simulink model "main_sim5"  (R2023a)
settings: Solver=FixedStepAuto  StartTime=0.0  StopTime=T  FixedStep=dt  RelTol=1e-3
values from neighbouring files (symbols this model uses):
  A = -a * eye(4)    [main_real4_slx.m]    (also in main_sim5_slx.m)
  ctrl_dt = 2e-3    (= 0.002)    [main_real4_slx.m]    (also in main_sim5_slx.m = 0.001)
  dt = time(2) - time(1)    [check_PE_from_logsout.m]    (also in main_real4_slx.m = 0.002; main_sim5_slx.m = 0.001)
  eta1 = 1e3    (= 1000)    [main_real4_slx.m]    (also in main_sim5_slx.m = 0.1)
  eta2 = 1e2    (= 100)    [main_real4_slx.m]    (also in main_sim5_slx.m)
  Kd = [20 0 ... (first row only)    [main_real4_slx.m]    (also in main_sim5_slx.m)
  Kp = [100 0 ... (first row only)    [main_real4_slx.m]    (also in main_sim5_slx.m)
  N = length(time)    [check_PE_from_logsout.m]    (also in main_plotter5_1.m = length(X3); main_plotter5_2.m = length(X3))
  n_h = 100    [main_real4_slx.m]    (also in main_sim5_slx.m = 20)
  n_i = 6    [main_real4_slx.m]    (also in main_sim5_slx.m)
  n_o = 4    [main_real4_slx.m]    (also in main_sim5_slx.m)
  params = struct(     'm1', 2.465,     'm2', 2.465,     'l1', 0.2,     'l2', 0.2,     'lc1', 0.13888,     'lc2', 0.13888,     'I1', 0.06911,     'I2', 0.06911,     'I1m', 9*9*1002e-7,     'I2m', 9*9*1002e-7,     'b1', 0.5,     'b2', 0.7,     'fc1', 0.1,     'fc2', 0.1,     'k1', 1500,     'k2', 1500)    [main_real4_slx.m]    (also in main_sim5_slx.m = struct(     'm1', 2.465,     'm2', 2.465,     'l1', 0.2,    )
  rho1 = 0.0    (= 0)    [main_real4_slx.m]    (also in main_sim5_slx.m)
  rho2 = 0.0    (= 0)    [main_real4_slx.m]    (also in main_sim5_slx.m)
  V0 = 1e-2 * randn(n_h,n_i) + 0    [main_real4_slx.m]    (also in main_sim5_slx.m = 1e-1 * randn(n_h,n_i))
  W0 = 1e-2 * randn(n_o,n_h) + 0    [main_real4_slx.m]    (also in main_sim5_slx.m = 1e-1 * randn(n_o,n_h))
  X0 = [data_2901(1,1);data_2902(1,1);data_2901(2,1);data_2902(2,1)]    [main_real4_slx.m]    (also in main_sim5_slx.m = [-pi/2; 0; 0; 0])
  X_hat_0 = X0    [main_real4_slx.m]    (also in main_sim5_slx.m)
undefined symbols (not defined in the file or in its folder): I1, I1m, I2, I2m, J_V_t_buffer, J_W_t_buffer, l1, l2, lc1, lc2, m1, m2
settings Model: Creator=dding  LastModifiedBy=fairytale

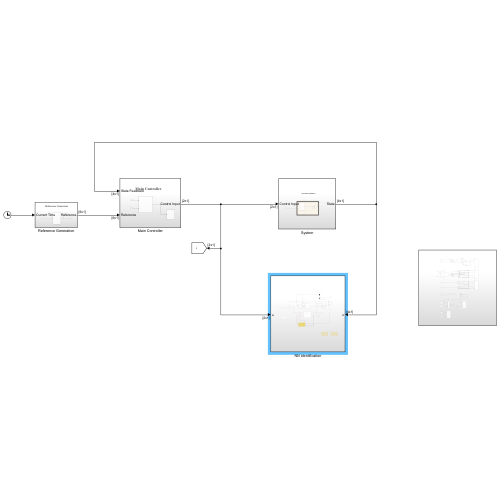
[thumbnail: Simulink's stored preview of the top-level diagram]
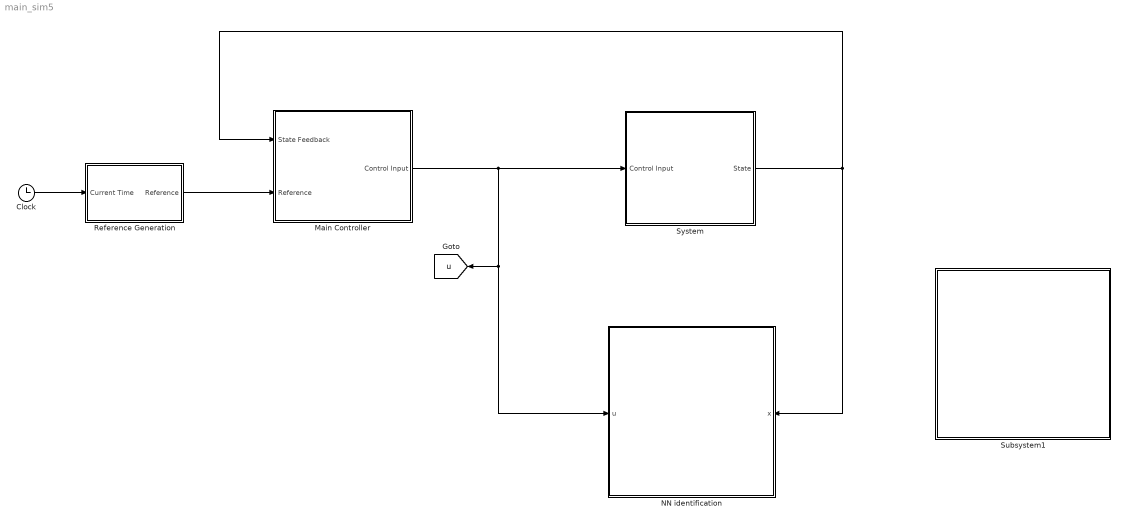
== system main_sim5 ==
  Clock : Clock
  Main Controller : Subsystem
  NN identification : Subsystem
      settings: PortSchema="{\"entries\":[{\"content\":{\"sides\":[{\"content\":{},\"type\":\"ConnectorPlacement.EquallySpacedRectSide\",\"uuid\":\"b5e68509-af14-483e-9022-a238da7f8976\"},{\"content\":{\"side\":\"RIGHT\"},\"type\":\"ConnectorPlacement.EquallySpacedRectSide\",\"uuid\":\"227b12d5-85c0-4871-b1f3-ce700a25cbd8\"},{\"content\":{\"connectorIds\":[\"In1\"],\"side\":\"TOP\"},\"type\":\"ConnectorPlacement.EquallySpacedRectSide\",\"uuid\":\"04532d91-bd13-4081-a0a6-2e9b5f5bbbc1\"},{\"content\":{\"connectorIds\":[\"In2\"],\"side\":\"BOTTOM\"},\"type\":\"ConnectorPlacement.EquallySpacedRectSide\",\"uuid\":\"58e23698-c698-43c7-afbb-9eb032c0630e\"}]},\"type\":\"ConnectorPlacement.EquallySpacedConnector\",\"uuid\":\"69e78e49-5ac8-44ff-82c8-e58de664d9c5\"}],\"packageUris\":[\"http://schema.mathworks.com/mf0/Connector/R2020b\"],\"version\":\"1.0\"}"
  Reference Generation : Subsystem
  Subsystem1 : Subsystem
  System : Subsystem
  tag scope: u=global
  wires:
  Reference Generation/1(Reference) -> Main Controller/2(Reference)
  Clock/1 -> Reference Generation/1(Current Time)
  Main Controller/1(Control Input) -> System/1(Control Input), NN identification/1(u), [u]
  System/1(State) -> NN identification/2(x), Main Controller/1(State Feedback)

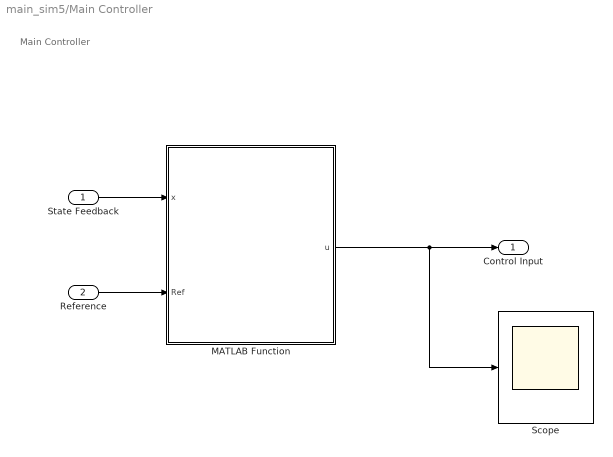
== system main_sim5/Main Controller ==
  note: Main Controller
  State Feedback : Inport
  Reference : Inport  Port=2
  MATLAB Function : MATLAB Function  TreatAsAtomicUnit=on  SystemSampleTime=ctrl_dt
  Scope : Scope
  Control Input : Outport
  wires:
  Reference/1 -> MATLAB Function/2(Ref)
  State Feedback/1 -> MATLAB Function/1(x)
  MATLAB Function/1(u) -> Scope/1, Control Input/1

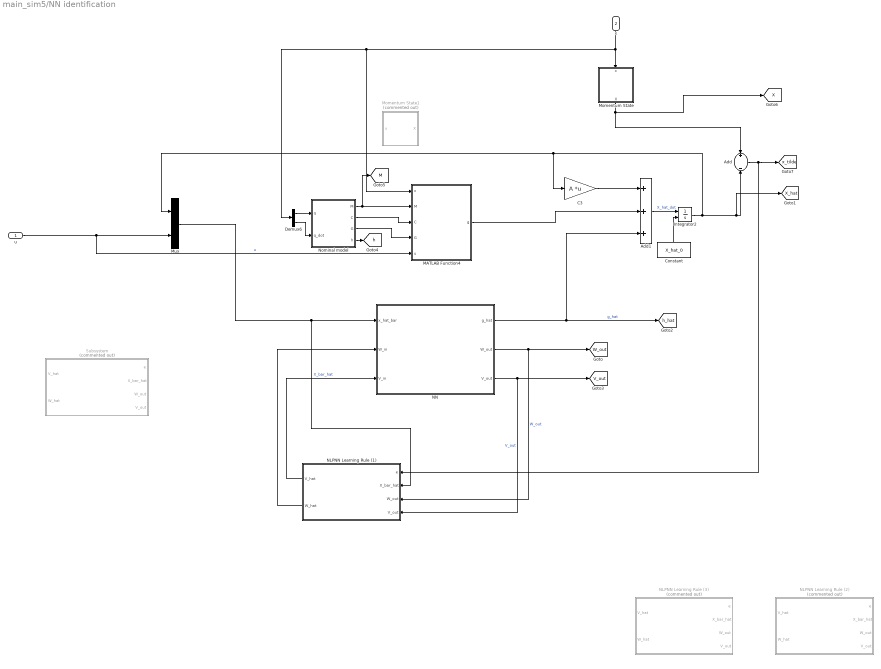
== system main_sim5/NN identification ==
  u : Inport
  x : Inport  Port=2
  Add : Sum  Inputs=+-
  Add1 : Sum  Inputs=+++
  C3 : Gain  Gain=A  Multiplication=Matrix(K*u)
  Constant : Constant  Value=X_hat_0  VectorParams1D=off
  Demux6 : Demux  Outputs=2
  Integrator2 : Integrator  InitialConditionSource=external  InitialCondition=X_hat_0
  MATLAB Function4 : MATLAB Function  TreatAsAtomicUnit=on
  Momentum State : MATLAB Function  TreatAsAtomicUnit=on
  Momentum State1 : MATLAB Function  Commented=on  TreatAsAtomicUnit=on
  Mux : Mux  Inputs=2
  NLPNN Learning Rule (1) : Subsystem
  NLPNN Learning Rule (2) : Subsystem  Commented=on
  NLPNN Learning Rule (3) : Subsystem  Commented=on
  NN : MATLAB Function  TreatAsAtomicUnit=on
  Nominal model : MATLAB Function  TreatAsAtomicUnit=on
  Subsystem : Subsystem  Commented=on
  tag scope: M=global, V_out=global, W_out=global, X=global, X_hat=global, h=global, h_hat=global, x_tilde=global
  wires:
  x/1 -> Demux6/1, MATLAB Function4/1(x), Momentum State/1(x)
  NN/2(W_out) -> NLPNN Learning Rule (1)/3(W_out), [W_out]  "W_out"
  Integrator2/1 -> Add/2, [X_hat], C3/1, Mux/1
  Add1/1 -> Integrator2/1  "X_hat_dot"
  NN/3(V_out) -> NLPNN Learning Rule (1)/4(V_out), [V_out]  "V_out"
  u/1 -> MATLAB Function4/5(u), Mux/2  "u"
  C3/1 -> Add1/1
  NN/1(g_hat) -> [h_hat], Add1/3  "g_hat"
  Constant/1 -> Integrator2/2
  Mux/1 -> NLPNN Learning Rule (1)/2(X_bar_hat), NN/1(x_hat_bar)  "X_bar_hat"
  Demux6/1 -> Nominal model/1(q)
  Nominal model/1(M) -> MATLAB Function4/2(M), [M]
  Nominal model/3(G) -> MATLAB Function4/4(G)
  Nominal model/2(C) -> MATLAB Function4/3(C)
  Demux6/2 -> Nominal model/2(q_dot)
  Momentum State/1(X) -> [X], Add/1
  Nominal model/4(h) -> [h]
  Add/1 -> NLPNN Learning Rule (1)/1(e), [x_tilde]
  NLPNN Learning Rule (1)/1(V_hat) -> NN/3(V_in)
  NLPNN Learning Rule (1)/2(W_hat) -> NN/2(W_in)
  MATLAB Function4/1(g) -> Add1/2

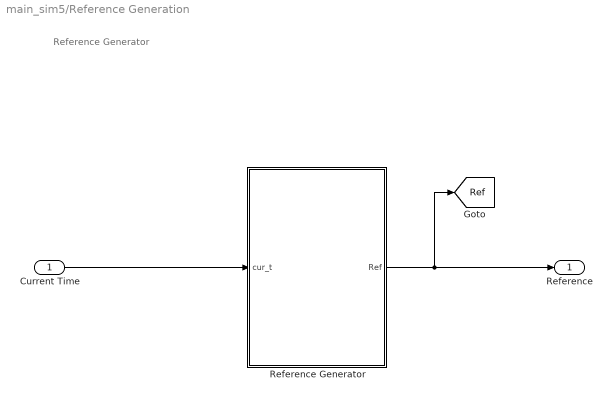
== system main_sim5/Reference Generation ==
  note: Reference Generator
  Current Time : Inport
  Reference Generator : MATLAB Function  TreatAsAtomicUnit=on
  Reference : Outport
  tag scope: Ref=global
  wires:
  Current Time/1 -> Reference Generator/1(cur_t)
  Reference Generator/1(Ref) -> [Ref], Reference/1

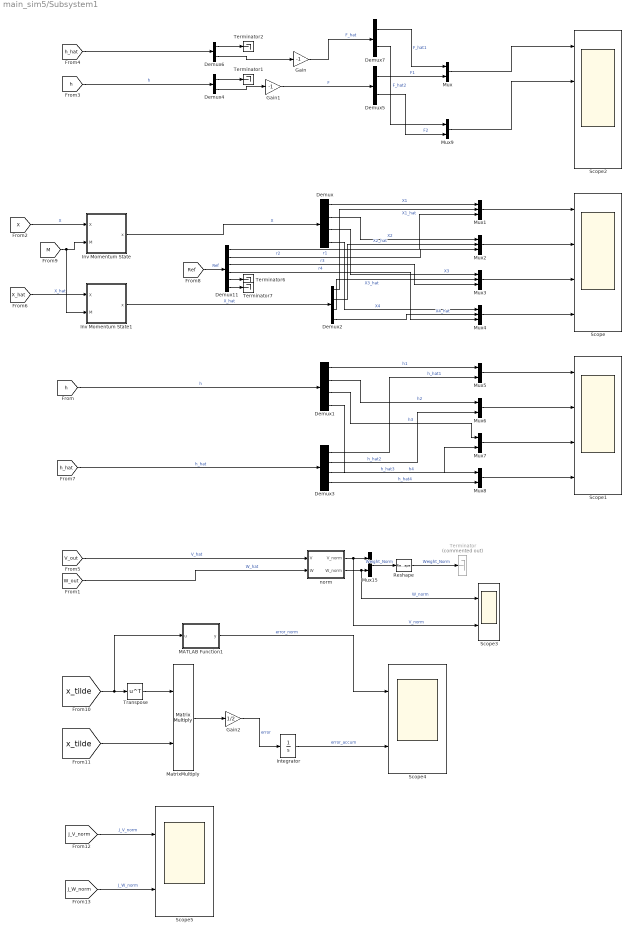
== system main_sim5/Subsystem1 ==
  Demux{,1..3} (4 alike) : Demux
  Demux11 : Demux  Outputs=6
  Demux{4..7} (4 alike) : Demux  Outputs=2
  Gain : Gain  Gain=-1
  Gain1 : Gain  Gain=-1
  Gain2 : Gain  Gain=1/2
  Integrator : Integrator
  Inv Momentum State : MATLAB Function  TreatAsAtomicUnit=on
  Inv Momentum State1 : MATLAB Function  TreatAsAtomicUnit=on
  MATLAB Function1 : MATLAB Function  TreatAsAtomicUnit=on
  MatrixMultiply : Product  Multiplication=Matrix(*)
  Mux{,5..9,15} (7 alike) : Mux  Inputs=2
  Mux{1..4} (4 alike) : Mux  Inputs=3
  Reshape : Reshape  OutputDimensionality=Column vector (2-D)
  Scope : Scope  NumInputPorts=4
  Scope1 : Scope  NumInputPorts=4
  Scope2 : Scope  NumInputPorts=4
  Scope3 : Scope  NumInputPorts=2
  Scope4 : Scope  NumInputPorts=2
  Scope5 : Scope  NumInputPorts=2
  Terminator : Terminator  Commented=on
  Terminator{1..2,6..7} (4 alike) : Terminator
  Transpose : Math  Operator=transpose
  norm : MATLAB Function  TreatAsAtomicUnit=on
  wires:
  Demux2/2 -> Mux2/2  "X2_hat"
  Mux4/1 -> Scope/4
  Demux1/4 -> Mux8/1  "h4"
  Mux3/1 -> Scope/3
  [h_hat] -> Demux3/1  "h_hat"
  Demux3/1 -> Mux5/2  "h_hat1"
  Demux3/2 -> Mux6/2  "h_hat2"
  Demux/1 -> Mux1/1  "X1"
  [Ref] -> Demux11/1  "Ref"
  Mux5/1 -> Scope1/1
  Demux1/1 -> Mux5/1  "h1"
  Mux2/1 -> Scope/2
  Demux2/4 -> Mux4/2  "X4_hat"
  Demux/3 -> Mux3/1  "X3"
  Demux11/1 -> Mux1/3  "r1"
  Mux6/1 -> Scope1/2
  Demux11/3 -> Mux3/3  "r3"
  Demux11/2 -> Mux2/3  "r2"
  Mux7/1 -> Scope1/3
  Demux2/1 -> Mux1/2  "X1_hat"
  Mux8/1 -> Scope1/4
  Demux2/3 -> Mux3/2  "X3_hat"
  Demux/4 -> Mux4/1  "X4"
  Demux11/6 -> Terminator7/1
  Demux/2 -> Mux2/1  "X2"
  Mux1/1 -> Scope/1
  Demux3/4 -> Mux8/2  "h_hat4"
  Demux11/5 -> Terminator6/1
  [h_hat] -> Demux6/1
  Demux1/2 -> Mux6/1  "h2"
  Demux3/3 -> Mux7/2  "h_hat3"
  Demux1/3 -> Mux7/1  "h3"
  [h] -> Demux1/1  "h"
  Demux11/4 -> Mux4/3  "r4"
  Demux5/1 -> Mux/2  "F1"
  Demux5/2 -> Mux9/2  "F2"
  norm/1(V_norm) -> Scope3/2, Mux15/1  "V_norm"
  Reshape/1 -> Terminator/1  "Weight_Norm"
  norm/2(W_norm) -> Scope3/1, Mux15/2  "W_norm"
  Mux15/1 -> Reshape/1  "Weight_Norm"
  [W_out] -> norm/2(W)  "W_hat"
  [V_out] -> norm/1(V)  "V_hat"
  [h] -> Demux4/1  "h"
  Demux4/1 -> Terminator1/1
  Demux6/1 -> Terminator2/1
  Demux6/2 -> Gain/1
  Demux4/2 -> Gain1/1
  Gain1/1 -> Demux5/1  "F"
  Gain/1 -> Demux7/1  "F_hat"
  Demux7/1 -> Mux/1  "F_hat1"
  Demux7/2 -> Mux9/1  "F_hat2"
  Mux/1 -> Scope2/1
  Mux9/1 -> Scope2/2
  [X] -> Inv Momentum State/1(X)  "X"
  [X_hat] -> Inv Momentum State1/1(X)  "X_hat"
  Inv Momentum State/1(x) -> Demux/1  "X"
  Inv Momentum State1/1(x) -> Demux2/1  "X_hat"
  [M] -> Inv Momentum State1/2(M), Inv Momentum State/2(M)
  [x_tilde] -> MATLAB Function1/1(u), Transpose/1
  Transpose/1 -> MatrixMultiply/1
  [x_tilde] -> MatrixMultiply/2
  MatrixMultiply/1 -> Gain2/1
  Gain2/1 -> Integrator/1  "error"
  Integrator/1 -> Scope4/2  "error_accum"
  [J_V_norm] -> Scope5/1  "J_V_norm"
  [J_W_norm] -> Scope5/2  "J_W_norm"
  MATLAB Function1/1(y) -> Scope4/1  "error_norm"

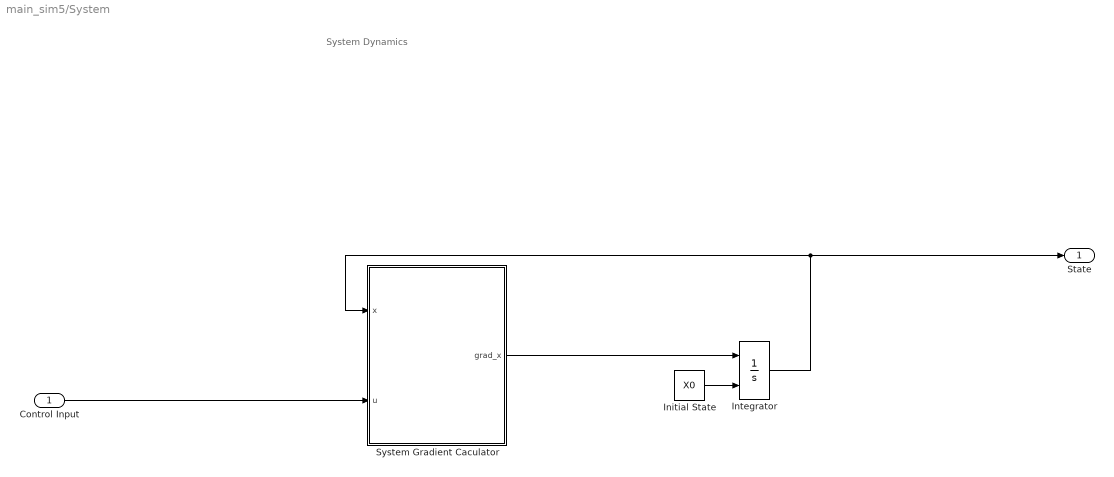
== system main_sim5/System ==
  note: System Dynamics
  Control Input : Inport
  Initial State : Constant  Value=X0  VectorParams1D=off
  Integrator : Integrator  InitialConditionSource=external
  System Gradient Caculator : MATLAB Function  TreatAsAtomicUnit=on
  State : Outport
  wires:
  Initial State/1 -> Integrator/2
  Control Input/1 -> System Gradient Caculator/2(u)
  Integrator/1 -> System Gradient Caculator/1(x), State/1
  System Gradient Caculator/1(grad_x) -> Integrator/1

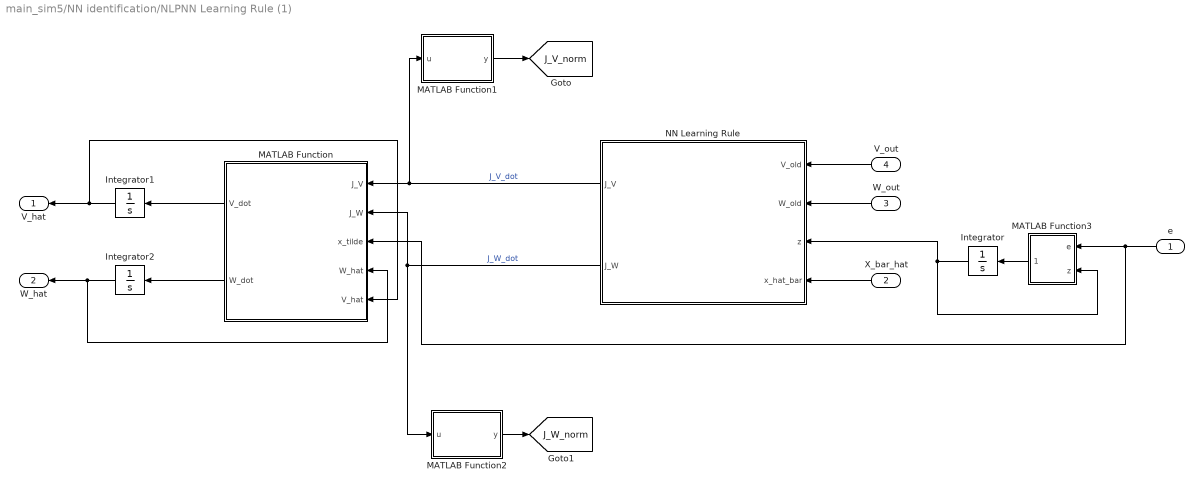
== system main_sim5/NN identification/NLPNN Learning Rule (1) ==
  e : Inport
  X_bar_hat : Inport  Port=2
  W_out : Inport  Port=3
  V_out : Inport  Port=4
  Integrator : Integrator  InitialCondition=[0,0,0,0]'
  Integrator1 : Integrator  InitialCondition=V0
  Integrator2 : Integrator  InitialCondition=W0
  MATLAB Function : MATLAB Function  TreatAsAtomicUnit=on
  MATLAB Function1 : MATLAB Function  TreatAsAtomicUnit=on
  MATLAB Function2 : MATLAB Function  TreatAsAtomicUnit=on
  MATLAB Function3 : MATLAB Function  TreatAsAtomicUnit=on
  NN Learning Rule : MATLAB Function  TreatAsAtomicUnit=on
  V_hat : Outport
  W_hat : Outport  Port=2
  tag scope: J_V_norm=global, J_W_norm=global
  wires:
  e/1 -> MATLAB Function/3(x_tilde), MATLAB Function3/1(e)
  X_bar_hat/1 -> NN Learning Rule/4(x_hat_bar)
  W_out/1 -> NN Learning Rule/2(W_old)
  V_out/1 -> NN Learning Rule/1(V_old)
  MATLAB Function/1(V_dot) -> Integrator1/1
  Integrator1/1 -> MATLAB Function/5(V_hat), V_hat/1
  Integrator2/1 -> MATLAB Function/4(W_hat), W_hat/1
  MATLAB Function/2(W_dot) -> Integrator2/1
  MATLAB Function1/1(y) -> [J_V_norm]
  MATLAB Function2/1(y) -> [J_W_norm]
  MATLAB Function3/1(z_dot) -> Integrator/1
  NN Learning Rule/2(J_W) -> MATLAB Function2/1(u), MATLAB Function/2(J_W)  "J_W_dot"
  NN Learning Rule/1(J_V) -> MATLAB Function1/1(u), MATLAB Function/1(J_V)  "J_V_dot"
  Integrator/1 -> MATLAB Function3/2(z), NN Learning Rule/3(z)

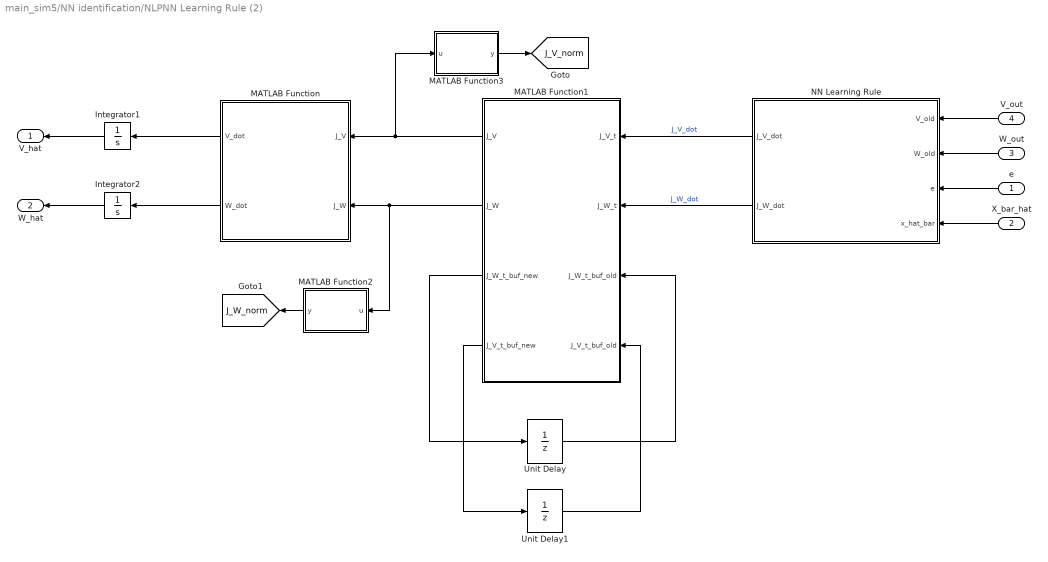
== system main_sim5/NN identification/NLPNN Learning Rule (2) ==
  e : Inport
  X_bar_hat : Inport  Port=2
  W_out : Inport  Port=3
  V_out : Inport  Port=4
  Integrator1 : Integrator  InitialCondition=V0
  Integrator2 : Integrator  InitialCondition=W0
  MATLAB Function : MATLAB Function  TreatAsAtomicUnit=on
  MATLAB Function1 : MATLAB Function  TreatAsAtomicUnit=on
  MATLAB Function2 : MATLAB Function  TreatAsAtomicUnit=on
  MATLAB Function3 : MATLAB Function  TreatAsAtomicUnit=on
  NN Learning Rule : MATLAB Function  TreatAsAtomicUnit=on
  Unit Delay : UnitDelay  InitialCondition=J_W_t_buffer  SampleTime=-1  HasFrameUpgradeWarning=on
  Unit Delay1 : UnitDelay  InitialCondition=J_V_t_buffer  SampleTime=-1  HasFrameUpgradeWarning=on
  V_hat : Outport
  W_hat : Outport  Port=2
  tag scope: J_V_norm=global, J_W_norm=global
  wires:
  e/1 -> NN Learning Rule/3(e)
  X_bar_hat/1 -> NN Learning Rule/4(x_hat_bar)
  W_out/1 -> NN Learning Rule/2(W_old)
  V_out/1 -> NN Learning Rule/1(V_old)
  NN Learning Rule/1(J_V_dot) -> MATLAB Function1/1(J_V_t)  "J_V_dot"
  NN Learning Rule/2(J_W_dot) -> MATLAB Function1/2(J_W_t)  "J_W_dot"
  MATLAB Function/1(V_dot) -> Integrator1/1
  Integrator1/1 -> V_hat/1
  Integrator2/1 -> W_hat/1
  MATLAB Function/2(W_dot) -> Integrator2/1
  MATLAB Function1/1(J_V) -> MATLAB Function3/1(u), MATLAB Function/1(J_V)
  MATLAB Function1/2(J_W) -> MATLAB Function2/1(u), MATLAB Function/2(J_W)
  Unit Delay/1 -> MATLAB Function1/3(J_W_t_buf_old)
  MATLAB Function1/3(J_W_t_buf_new) -> Unit Delay/1
  MATLAB Function1/4(J_V_t_buf_new) -> Unit Delay1/1
  Unit Delay1/1 -> MATLAB Function1/4(J_V_t_buf_old)
  MATLAB Function2/1(y) -> [J_W_norm]
  MATLAB Function3/1(y) -> [J_V_norm]

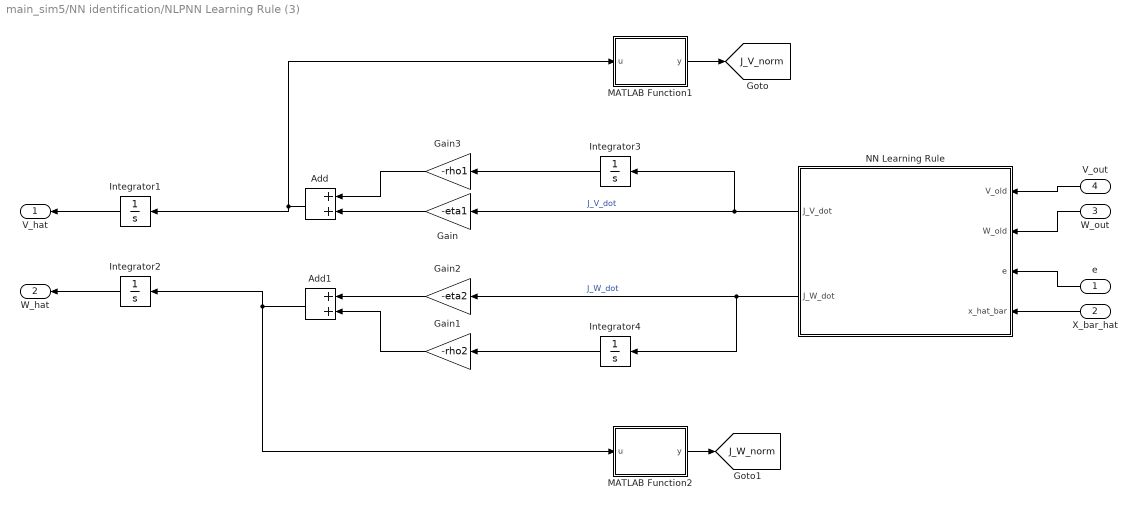
== system main_sim5/NN identification/NLPNN Learning Rule (3) ==
  e : Inport
  X_bar_hat : Inport  Port=2
  W_out : Inport  Port=3
  V_out : Inport  Port=4
  Add : Sum
  Add1 : Sum
  Gain : Gain  Gain=-eta1
  Gain1 : Gain  Gain=-rho2
  Gain2 : Gain  Gain=-eta2
  Gain3 : Gain  Gain=-rho1
  Integrator1 : Integrator  InitialCondition=V0
  Integrator2 : Integrator  InitialCondition=W0
  Integrator3 : Integrator  InitialCondition=zeros(n_h,n_i)
  Integrator4 : Integrator  InitialCondition=zeros(n_o,n_h)
  MATLAB Function1 : MATLAB Function  TreatAsAtomicUnit=on
  MATLAB Function2 : MATLAB Function  TreatAsAtomicUnit=on
  NN Learning Rule : MATLAB Function  TreatAsAtomicUnit=on
  V_hat : Outport
  W_hat : Outport  Port=2
  tag scope: J_V_norm=global, J_W_norm=global
  wires:
  Integrator4/1 -> Gain1/1
  e/1 -> NN Learning Rule/3(e)
  X_bar_hat/1 -> NN Learning Rule/4(x_hat_bar)
  W_out/1 -> NN Learning Rule/2(W_old)
  V_out/1 -> NN Learning Rule/1(V_old)
  NN Learning Rule/1(J_V_dot) -> Gain/1, Integrator3/1  "J_V_dot"
  NN Learning Rule/2(J_W_dot) -> Gain2/1, Integrator4/1  "J_W_dot"
  Integrator1/1 -> V_hat/1
  Integrator2/1 -> W_hat/1
  MATLAB Function1/1(y) -> [J_V_norm]
  MATLAB Function2/1(y) -> [J_W_norm]
  Add/1 -> MATLAB Function1/1(u), Integrator1/1
  Add1/1 -> Integrator2/1, MATLAB Function2/1(u)
  Gain/1 -> Add/2
  Gain2/1 -> Add1/1
  Gain1/1 -> Add1/2
  Integrator3/1 -> Gain3/1
  Gain3/1 -> Add/1

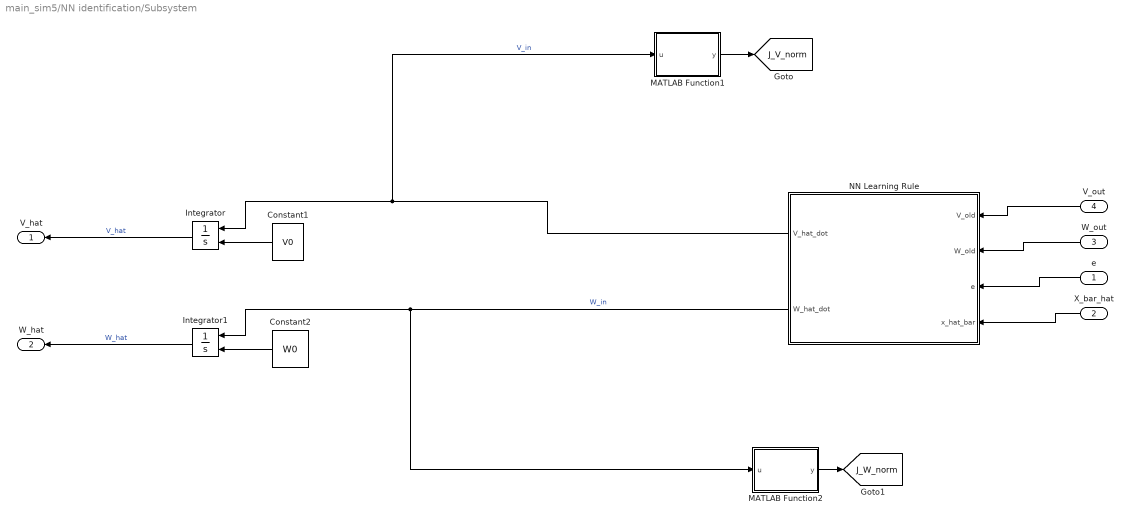
== system main_sim5/NN identification/Subsystem ==
  e : Inport
  X_bar_hat : Inport  Port=2
  W_out : Inport  Port=3
  V_out : Inport  Port=4
  Constant1 : Constant  Value=V0  VectorParams1D=off
  Constant2 : Constant  Value=W0  VectorParams1D=off
  Integrator : Integrator  InitialConditionSource=external  InitialCondition=V0
  Integrator1 : Integrator  InitialConditionSource=external  InitialCondition=W0
  MATLAB Function1 : MATLAB Function  TreatAsAtomicUnit=on
  MATLAB Function2 : MATLAB Function  TreatAsAtomicUnit=on
  NN Learning Rule : MATLAB Function  TreatAsAtomicUnit=on
  V_hat : Outport
  W_hat : Outport  Port=2
  tag scope: J_V_norm=global, J_W_norm=global
  wires:
  Constant2/1 -> Integrator1/2
  Constant1/1 -> Integrator/2
  Integrator/1 -> V_hat/1  "V_hat"
  e/1 -> NN Learning Rule/3(e)
  Integrator1/1 -> W_hat/1  "W_hat"
  W_out/1 -> NN Learning Rule/2(W_old)
  X_bar_hat/1 -> NN Learning Rule/4(x_hat_bar)
  V_out/1 -> NN Learning Rule/1(V_old)
  NN Learning Rule/1(V_hat_dot) -> MATLAB Function1/1(u), Integrator/1  "V_in"
  NN Learning Rule/2(W_hat_dot) -> MATLAB Function2/1(u), Integrator1/1  "W_in"
  MATLAB Function1/1(y) -> [J_V_norm]
  MATLAB Function2/1(y) -> [J_W_norm]

== matlab function main_sim5/Reference Generation/Reference Generator ==
  data: cur_t input size=1; Ref output size=[6 1]; Traj_flag parameter
function Ref = ref_gen_trajectory_based(cur_t, Traj_flag)
    % Set waypoints and parameters based on Traj_flag

    if Traj_flag == 1
        % === Trajectory 1 ===
        q0 = [-pi/2; 0];
        qd1 = [pi/4; pi/2];
        qd2 = [pi/4 + pi/2; -pi/2];
        % waypoints = [q0, ... 
        %      qd1, qd3, qd1, qd4, qd3, qd1, qd2, qd3, qd2, qd1, ...
        %      qd3, qd2, qd4, qd2, qd1, qd3, qd4, qd1, qd3, qd2, ...
        %      qd1, q0];
        waypoints = [q0, ... 
                     qd1, qd2, qd1, qd2, qd1, qd2, qd1, qd2, qd1, qd2, ...
                     qd1, qd2, qd1, qd2, qd1, qd2, qd1, qd2, qd1, qd2, ...
                     qd1, q0];
        traj_duration = 4.0;
        init_duration = 4.0;
        end_duration = 4.0;
    else
        % === Trajectory 2 ===
        q0 = [-pi/2; 0];
        qd1 = [-pi/3; 2*pi/3];
        qd2 = [pi/3; -2*pi/3];
        waypoints = [q0, ... 
                     qd1, qd2, qd1, qd2, qd1, qd2, qd1, qd2, qd1, qd2, ...
                     qd1, qd2, qd1, qd2, qd1, qd2, qd1, qd2, qd1, qd2, ...
                     qd1, q0];
        traj_duration = 20.0;
        init_duration = 4.0;
        end_duration = 4.0;
    end
    
    % === 공통 처리 ===
    num_segments = size(waypoints, 2) - 1;
    
    traj_times = traj_duration * ones(1, num_segments);
    traj_times(1) = init_duration;
    traj_times(end) = end_duration;
    
    Tidle = 0;

    % Compute total time
    Ttotal = Tidle * (num_segments + 1) + sum(traj_times);

    if cur_t >= Ttotal
        Ref = [waypoints(:,end); zeros(4,1)]; % stop
        return;
    end

    
    % Initial idle
    if cur_t < Tidle
        Ref = [waypoints(:,1); zeros(4,1)];
        return;
    end
    t_marker = Tidle;

    % Segment + idle loop
    for i = 1:num_segments
        % Trajectory segment
        if cur_t < t_marker + traj_times(i)
            t_local = cur_t - t_marker;
            Ref = poly_traj_5th(waypoints(:,i), waypoints(:,i+1), traj_times(i), t_local);
            return;
        end
        t_marker = t_marker + traj_times(i);

        % Idle after segment
        if cur_t < t_marker + Tidle
            Ref = [waypoints(:,i+1); zeros(4,1)];
            return;
        end
        t_marker = t_marker + Tidle;
    end
    Ref = [waypoints(:,end); zeros(4,1)];

end

function poly5 = poly_traj_5th(r0, rf, T, t)
    D = rf - r0;
    a0 = r0;
    a1 = 0;
    a2 = 0;
    a3 = 10 * D / T^3;
    a4 = -15 * D / T^4;
    a5 = 6 * D / T^5;

    r     = a0 + a1*t + a2*t^2 + a3*t^3 + a4*t^4 + a5*t^5;
    rdot  = a1 + 2*a2*t + 3*a3*t^2 + 4*a4*t^3 + 5*a5*t^4;
    rddot = 2*a2 + 6*a3*t + 12*a4*t^2 + 20*a5*t^3;

    poly5 = [r; rdot; rddot];
end


% function Ref = ref_gen(Ref_i, Ref_f, cur_t, T, index, repeat_n)
% 
%     % 5th order Polynomial trajectory 
%     t0 = 0; tf = T; % Start and end times
% 
%     ri = Ref_i(1:2);
%     rdoti = Ref_i(3:4);
%     rddoti = Ref_i(5:6);
% 
%     rf = Ref_f(1:2);
%     rdotf = Ref_f(3:4);
%     rddotf = Ref_f(5:6);
% 
%     if index == 1
%         if cur_t > T
%             % After T, maintain final position, velocity, and acceleration
%             ref = rf;
%             ref_dot = rdotf;
%             ref_ddot = rddotf; % Final acceleration is zero
%             Ref = [ref;ref_dot;ref_ddot];
%         else
%             % Solve for coefficients for each dimension
%             A = [1, t0, t0^2, t0^3, t0^4, t0^5;         % ri
%                 0, 1,  2*t0, 3*t0^2, 4*t0^3, 5*t0^4;   % rdoti
%                 0, 0,  2,    6*t0, 12*t0^2, 20*t0^3;   % initial acceleration (0)
%                 1, tf, tf^2, tf^3, tf^4, tf^5;         % rf
%                 0, 1,  2*tf, 3*tf^2, 4*tf^3, 5*tf^4;   % rdotf
%                 0, 0,  2,    6*tf, 12*tf^2, 20*tf^3];  % final acceleration (0)
% 
%             coeff_x = A \ [ri(1); rdoti(1); 0; rf(1); rdotf(1); 0];
%             coeff_y = A \ [ri(2); rdoti(2); 0; rf(2); rdotf(2); 0];
% 
%             % Compute reference, its derivative, and second derivative
%             ref = [coeff_x(1) + coeff_x(2)*cur_t + coeff_x(3)*cur_t^2 + coeff_x(4)*cur_t^3 + coeff_x(5)*cur_t^4 + coeff_x(6)*cur_t^5;
%                 coeff_y(1) + coeff_y(2)*cur_t + coeff_y(3)*cur_t^2 + coeff_y(4)*cur_t^3 + coeff_y(5)*cur_t^4 + coeff_y(6)*cur_t^5];
%             ref_dot = [coeff_x(2) + 2*coeff_x(3)*cur_t + 3*coeff_x(4)*cur_t^2 + 4*coeff_x(5)*cur_t^3 + 5*coeff_x(6)*cur_t^4;
%                     coeff_y(2) + 2*coeff_y(3)*cur_t + 3*coeff_y(4)*cur_t^2 + 4*coeff_y(5)*cur_t^3 + 5*coeff_y(6)*cur_t^4];
%             ref_ddot = [2*coeff_x(3) + 6*coeff_x(4)*cur_t + 12*coeff_x(5)*cur_t^2 + 20*coeff_x(6)*cur_t^3;
%                         2*coeff_y(3) + 6*coeff_y(4)*cur_t + 12*coeff_y(5)*cur_t^2 + 20*coeff_y(6)*cur_t^3];
%             Ref = [ref;ref_dot;ref_ddot];
%         end
% 
%     %index == 2
%     else
%         total_T = repeat_n * T;
%         if cur_t > total_T
%             ref = ri;
%             ref_dot = rdoti;
%             ref_ddot = [0; 0];
% 
%             Ref = [ref;ref_dot;ref_ddot];
%             return;
%         end
% 
%         % 현재 몇 번째 사이클인지 (0부터 시작)
%         cycle_count = floor(cur_t / T);
%         t_in_cycle = cur_t - cycle_count * T;
% 
%         T1 = T/2; T2 = T/2;
% 
%         if t_in_cycle <= T1
%             % First segment: ri -> rf
%             seg_t = t_in_cycle;
%             seg_ri = ri;
%             seg_rdoti = rdoti;
%             seg_rf = rf;
%             seg_rdotf = [0; 0];
%             seg_T = T1;
%         else
%             % Second segment: rf -> ri
%             seg_t = t_in_cycle - T1;
%             seg_ri = rf;
%             seg_rdoti = [0; 0];
%             seg_rf = ri;
%             seg_rdotf = [0; 0];
%             seg_T = T2;
%         end
% 
%         % 5th order polynomial for each segment
%         t0 = 0; tf = seg_T;
%         A = [1, t0, t0^2, t0^3, t0^4, t0^5;
%              0, 1,  2*t0, 3*t0^2, 4*t0^3, 5*t0^4;
%              0, 0,  2,    6*t0, 12*t0^2, 20*t0^3;
%              1, tf, tf^2, tf^3, tf^4, tf^5;
%              0, 1,  2*tf, 3*tf^2, 4*tf^3, 5*tf^4;
%              0, 0,  2,    6*tf, 12*tf^2, 20*tf^3];
% 
%         coeff_x = A \ [seg_ri(1); seg_rdoti(1); 0; seg_rf(1); seg_rdotf(1); 0];
%         coeff_y = A \ [seg_ri(2); seg_rdoti(2); 0; seg_rf(2); seg_rdotf(2); 0];
% 
%         ref = [coeff_x(1) + coeff_x(2)*seg_t + coeff_x(3)*seg_t^2 + coeff_x(4)*seg_t^3 + coeff_x(5)*seg_t^4 + coeff_x(6)*seg_t^5;
%                coeff_y(1) + coeff_y(2)*seg_t + coeff_y(3)*seg_t^2 + coeff_y(4)*seg_t^3 + coeff_y(5)*seg_t^4 + coeff_y(6)*seg_t^5];
%         ref_dot = [coeff_x(2) + 2*coeff_x(3)*seg_t + 3*coeff_x(4)*seg_t^2 + 4*coeff_x(5)*seg_t^3 + 5*coeff_x(6)*seg_t^4;
%                    coeff_y(2) + 2*coeff_y(3)*seg_t + 3*coeff_y(4)*seg_t^2 + 4*coeff_y(5)*seg_t^3 + 5*coeff_y(6)*seg_t^4];
%         ref_ddot = [2*coeff_x(3) + 6*coeff_x(4)*seg_t + 12*coeff_x(5)*seg_t^2 + 20*coeff_x(6)*seg_t^3;
%                     2*coeff_y(3) + 6*coeff_y(4)*seg_t + 12*coeff_y(5)*seg_t^2 + 20*coeff_y(6)*seg_t^3];
% 
%         Ref = [ref;ref_dot;ref_ddot];
% 
%         return;
%     end
% 
% end

== matlab function main_sim5/Subsystem1/norm ==
  data: V input; V_norm output; W_norm output; W input
function [V_norm,W_norm] = Norm(V, W)

    V_norm = norm(V,'fro');
    W_norm = norm(W, 'fro');
end

== matlab function main_sim5/Main Controller/MATLAB Function ==
  data: x input size=[4 1]; u output size=[2 1]; Ref input size=[6 1]; params parameter; Kp parameter; Kd parameter
function u = fcn(x, Ref, params, Kp, Kd)

    ref_q = Ref(1:2);
    ref_qdot = Ref(3:4);
    ref_qddot = Ref(5:6);

    e = ref_q - x(1:2);
    edot = ref_qdot - x(3:4);

    [M, C, G] = two_link_model(x(1:2), x(3:4), params);
    
    u = (M * (ref_qddot + Kp * e + Kd * edot) + C * x(3:4) + G);

end

function [M, C, G] = two_link_model(q, q_dot, params)
%%
    m1 = params.m1;  m2 = params.m2;
    l1 = params.l1;  l2 = params.l2;
    lc1 = params.lc1;  lc2 = params.lc2;
    I1 = params.I1;  I2 = params.I2;
    I1m = params.I1m; I2m = params.I2m;
    b1 = params.b1;  b2 = params.b2;
    fc1 = params.fc1; fc2 = params.fc2;
    k1 = params.k1;  k2 = params.k2;
    %%
    q1 = q(1); q2 = q(2);
    q_dot1 = q_dot(1); q_dot2 = q_dot(2); 
  
    g = 9.81;    
    %%
    Mmat11=I1+I2+lc1^2*m1+l1^2*m2+lc2^2*m2+2*l1*lc2*m2*cos(q2);
    Mmat12=I2+lc2^2*m2+l1*lc2*m2*cos(q2);
    Mmat21=I2+lc2^2*m2+l1*lc2*m2*cos(q2);
    Mmat22=I2+lc2^2*m2;
    
    Cmat11=(-1)*l1*lc2*m2*sin(q2)*q_dot2;
    Cmat12=(-1)*l1*lc2*m2*sin(q2)*(q_dot1+q_dot2);
    Cmat21=l1.*lc2*m2*sin(q2)*q_dot1;
    Cmat22=0;
    
    Gmat1=g*((lc1*m1+l1*m2)*cos(q1)+lc2*m2*cos(q1+q2));
    Gmat2=g*lc2*m2*cos(q1+q2);
    
    
    
    %%
    M = [
        Mmat11 Mmat12
        Mmat21 Mmat22  
        ];
    C = [
        Cmat11 Cmat12
        Cmat21 Cmat22  
        ];
    G = [
        Gmat1
        Gmat2
        ];

end

== matlab function main_sim5/System/System Gradient Caculator ==
  data: x input size=[4 1]; u input size=[2 1]; grad_x output; params parameter
function grad_x = fcn(x, u, params)

   [M, C, G, F] = two_link_model (x(1:2), x(3:4),params);


   grad_x =  [x(3:4) ; M \ (u - C * x(3:4) - G - F)];

end



function [M, C, G, F] = two_link_model(q, q_dot, params)
%%
    m1 = params.m1;  m2 = params.m2;
    l1 = params.l1;  l2 = params.l2;
    lc1 = params.lc1;  lc2 = params.lc2;
    I1 = params.I1;  I2 = params.I2;
    I1m = params.I1m; I2m = params.I2m;
    b1 = params.b1;  b2 = params.b2;
    fc1 = params.fc1; fc2 = params.fc2;
    k1 = params.k1;  k2 = params.k2;
    %%
    q1 = q(1); q2 = q(2);
    q_dot1 = q_dot(1); q_dot2 = q_dot(2); 
  
    g = 9.81;    
    %%
    Mmat11=I1+I2+lc1^2*m1+l1^2*m2+lc2^2*m2+2*l1*lc2*m2*cos(q2) + I1m;
    Mmat12=I2+lc2^2*m2+l1*lc2*m2*cos(q2);
    Mmat21=I2+lc2^2*m2+l1*lc2*m2*cos(q2);
    Mmat22=I2+lc2^2*m2+I2m;
    
    Cmat11=(-1)*l1*lc2*m2*sin(q2)*q_dot2;
    Cmat12=(-1)*l1*lc2*m2*sin(q2)*(q_dot1+q_dot2);
    Cmat21=l1.*lc2*m2*sin(q2)*q_dot1;
    Cmat22=0;
    
    Gmat1=g*((lc1*m1+l1*m2)*cos(q1)+lc2*m2*cos(q1+q2));
    Gmat2=g*lc2*m2*cos(q1+q2);
    
    
    Fmat1=b1*tanh(k1*q_dot1)+fc1*q_dot1;
    Fmat2=b2*tanh(k2*q_dot2)+fc2*q_dot2;
    
    
    %%
    M = [
        Mmat11 Mmat12
        Mmat21 Mmat22  
        ];
    C = [
        Cmat11 Cmat12
        Cmat21 Cmat22  
        ];
    G = [
        Gmat1
        Gmat2
        ];

    F = [
        Fmat1
        Fmat2
        ];   
    

end

== matlab function main_sim5/NN identification/MATLAB Function4 ==
  data: x input; M input; C input; G input; u input; g output; A parameter
function g = fcn(x,M,C,G,u,A)


    f = [x(3:4)
         C' * x(3:4) - G + u];

    X = [x(1:2)
         M * x(3:4)];

    g = f - A * X;

end

== matlab function main_sim5/NN identification/Nominal model ==
  data: q input; M output; C output; q_dot input; G output; params parameter; h output
function [M, C, G, h] = Nominal_model(q, q_dot, params)
    %%
    q1 = q(1); q2 = q(2);
    q_dot1 = q_dot(1); q_dot2 = q_dot(2); 
    
    m1 = params.m1;  m2 = params.m2;
    l1 = params.l1;  l2 = params.l2;
    lc1 = params.lc1;  lc2 = params.lc2;
    I1 = params.I1;  I2 = params.I2;
    I1m = params.I1m; I2m = params.I2m;
    b1 = params.b1;  b2 = params.b2;
    fc1 = params.fc1; fc2 = params.fc2;
    k1 = params.k1;  k2 = params.k2;

    g = 9.81;    
    %%
    Mmat11=I1+I2+lc1^2*m1+l1^2*m2+lc2^2*m2+2*l1*lc2*m2*cos(q2) + I1m;
    Mmat12=I2+lc2^2*m2+l1*lc2*m2*cos(q2);
    Mmat21=I2+lc2^2*m2+l1*lc2*m2*cos(q2);
    Mmat22=I2+lc2^2*m2 + I2m;
    
    Cmat11=(-1)*l1*lc2*m2*sin(q2)*q_dot2;
    Cmat12=(-1)*l1*lc2*m2*sin(q2)*(q_dot1+q_dot2);
    Cmat21=l1.*lc2*m2*sin(q2)*q_dot1;
    Cmat22=0;
    
    Gmat1=g*((lc1*m1+l1*m2)*cos(q1)+lc2*m2*cos(q1+q2));
    Gmat2=g*lc2*m2*cos(q1+q2);
    
    
    Fmat1=b1*tanh(k1*q_dot1)+fc1*q_dot1;
    Fmat2=b2*tanh(k2*q_dot2)+fc2*q_dot2;
    
    
    %%
    M = [
        Mmat11 Mmat12
        Mmat21 Mmat22  
        ];
    C = [
        Cmat11 Cmat12
        Cmat21 Cmat22  
        ];
    G = [
        Gmat1
        Gmat2
        ];

    F = [
        Fmat1
        Fmat2
        ];   

    h = [zeros(2,1);-F];

end

== matlab function main_sim5/NN identification/Subsystem/MATLAB Function1 ==
  data: u input; y output
function y = Norm(u)

y = norm(u,"fro");

== matlab function main_sim5/NN identification/Subsystem/MATLAB Function2 ==
  data: u input; y output
function y = Norm(u)

y = norm(u,"fro");

== matlab function main_sim5/NN identification/NLPNN Learning Rule (2)/MATLAB Function ==
  data: J_V input; V_dot output size=[n_h n_i]; J_W input; eta1 parameter; eta2 parameter; W_dot output size=[n_o n_h]
function [V_dot, W_dot] = fcn(J_V, J_W, eta1, eta2)


W_dot = - eta1 * J_W;
V_dot = - eta2 * J_V;

end

== matlab function main_sim5/NN identification/NLPNN Learning Rule (1)/MATLAB Function1 ==
  data: u input; y output
function y = Norm(u)

y = norm(u,"fro");

== matlab function main_sim5/NN identification/NLPNN Learning Rule (2)/NN Learning Rule ==
  data: J_V_dot output; J_W_dot output; V_old input; W_old input; e input; x_hat_bar input; A parameter; n_h parameter
function [J_V_dot, J_W_dot] = learningrule(V_old, W_old, e, x_hat_bar, A, n_h)

    % J = 1/2 * integral(x_tilde' * x_tilde * dt)
    W_hat = W_old;
    V_hat = V_old;

    % identification
    x_tilde = e;

    % Lambda = zeros(n_h,n_h);
    Lambda = diag(tanh(V_hat * x_hat_bar).^2);

    J_W_t = (x_tilde' * inv(A))' * activate(V_hat*x_hat_bar)';
    J_V_t = (x_tilde' * inv(A) * W_hat * (eye(size(Lambda)) - Lambda))' * x_hat_bar';
    
    J_W_dot = J_W_t;
    J_V_dot = J_V_t;
    
end

function sigma = activate(x)
    % sigma = tanh(x) + 2*ones(size(x));
    sigma = tanh(x);
end

== matlab function main_sim5/NN identification/NLPNN Learning Rule (1)/MATLAB Function2 ==
  data: u input; y output
function y = Norm(u)

y = norm(u,"fro");

== matlab function main_sim5/NN identification/NLPNN Learning Rule (1)/MATLAB Function ==
  data: J_V input; V_dot output size=[n_h n_i]; J_W input; eta1 parameter; eta2 parameter; W_dot output size=[n_o n_h]; x_tilde input; W_hat input; V_hat input; rho1 parameter; rho2 parameter
function [V_dot, W_dot] = fcn(J_V, J_W, eta1, eta2, x_tilde, W_hat, V_hat, rho1, rho2)


W_dot = - eta1 * J_W - rho1 * norm(x_tilde) * W_hat;
V_dot = - eta2 * J_V - rho2 * norm(x_tilde) * V_hat;

end

== matlab function main_sim5/NN identification/NLPNN Learning Rule (1)/NN Learning Rule ==
  data: J_V output; J_W output; V_old input; W_old input; z input; x_hat_bar input; A parameter; n_h parameter; rho1 parameter; rho2 parameter
function [J_V, J_W] = learningrule(V_old, W_old, z, x_hat_bar, A, n_h, rho1, rho2)

    % J = 1/2 * integral(x_tilde' * x_tilde * dt)
    W_hat = W_old;
    V_hat = V_old;
    

    % Lambda = zeros(n_h,n_h);
    Lambda = diag(tanh(V_hat * x_hat_bar).^2);

    % update the weights
    % W_hat_dot = - eta1 * (x_tilde' * inv(A))' * activate(V_hat*x_hat_bar)' - rho1 * norm(x_tilde) * W_hat;
    % V_hat_dot = - eta2 * (x_tilde' * inv(A) * W_hat * (eye(size(Lambda)) - Lambda))' * x_hat_bar' - rho2 * norm(x_tilde) * V_hat;
    


    J_W = (z' * inv(A))' * activate(V_hat*x_hat_bar)';
    J_V = (z' * inv(A) * W_hat * (eye(size(Lambda)) - Lambda))' * x_hat_bar';
    
end

function sigma = activate(x)
    % sigma = tanh(x) + 2*ones(size(x));
    sigma = tanh(x);
end

== matlab function main_sim5/Subsystem1/MATLAB Function1 ==
  data: u input; y output
function y = Norm(u)

y = norm(u,2);

== matlab function main_sim5/NN identification/NLPNN Learning Rule (2)/MATLAB Function1 ==
  settings: updateMethod=DISCRETE  sampleTime=dt
  data: J_V_t input; J_V output; J_W_t input; J_W_t_buf_old input; J_V_t_buf_old input; J_W output; dt parameter; n_h parameter; n_i parameter; N parameter; n_o parameter; J_W_t_buf_new output; J_V_t_buf_new output
function [J_V, J_W, J_W_t_buf_new, J_V_t_buf_new]  = update_gradient(J_V_t, J_W_t, J_W_t_buf_old, J_V_t_buf_old, dt, n_h, n_i, N, n_o)
    % % Constants
    n_o = 4;     % output dimension
    n_h = 100;   % hidden layer
    n_i = 6;     % input dimension
    % N   = 5;     % window size

    persistent idx
    if isempty(idx)
        idx = 1;
    end
    
    J_W_t_buffer = J_W_t_buf_old;
    J_V_t_buffer = J_V_t_buf_old;
    
    % === Reshape to column vectors ===
    J_W_vec = reshape(J_W_t, [], 1);   % (n_o * n_h × 1)
    J_V_vec = reshape(J_V_t, [], 1);   % (n_h * n_i × 1)
    
    % === Update sliding window buffers ===
    J_W_t_buffer(:, idx) = J_W_vec;
    J_V_t_buffer(:, idx) = J_V_vec;
    
    % === Advance index cyclically === 
    idx = mod(idx, N) + 1;
    
    % === Compute windowed average ===
    J_W_avg_vec = mean(J_W_t_buffer, 2);  % (n_o * n_h × 1)
    J_V_avg_vec = mean(J_V_t_buffer, 2);  % (n_h * n_i × 1)
    
    % === Reshape back to matrices ===
    J_W = reshape(J_W_avg_vec, n_o, n_h) * dt;
    J_V = reshape(J_V_avg_vec, n_h, n_i) * dt;

    J_W_t_buf_new = J_W_t_buffer;
    J_V_t_buf_new = J_V_t_buffer;

end

== matlab function main_sim5/NN identification/NLPNN Learning Rule (2)/MATLAB Function2 ==
  data: u input; y output
function y = Norm(u)

y = norm(u,"fro");

== matlab function main_sim5/NN identification/NLPNN Learning Rule (2)/MATLAB Function3 ==
  data: u input; y output
function y = Norm(u)

y = norm(u,"fro");

== matlab function main_sim5/NN identification/NLPNN Learning Rule (3)/MATLAB Function1 ==
  data: u input; y output
function y = Norm(u)

y = norm(u,"fro");

== matlab function main_sim5/NN identification/NLPNN Learning Rule (3)/MATLAB Function2 ==
  data: u input; y output
function y = Norm(u)

y = norm(u,"fro");

== matlab function main_sim5/NN identification/NLPNN Learning Rule (3)/NN Learning Rule ==
  data: J_V_dot output; J_W_dot output; V_old input; W_old input; e input; x_hat_bar input; A parameter; n_h parameter
function [J_V_dot, J_W_dot] = learningrule(V_old, W_old, e, x_hat_bar, A, n_h)

    % J = 1/2 * integral(x_tilde' * x_tilde * dt)
    W_hat = W_old;
    V_hat = V_old;
    % identification
    x_tilde = e;

    % Lambda = zeros(n_h,n_h);
    Lambda = diag(tanh(V_hat * x_hat_bar).^2);

    % update the weights
    % W_hat_dot = - eta1 * (x_tilde' * inv(A))' * activate(V_hat*x_hat_bar)' - rho1 * norm(x_tilde) * W_hat;
    % V_hat_dot = - eta2 * (x_tilde' * inv(A) * W_hat * (eye(size(Lambda)) - Lambda))' * x_hat_bar' - rho2 * norm(x_tilde) * V_hat;
    

    J_W_dot = (x_tilde' * inv(A))' * activate(V_hat*x_hat_bar)';
    J_V_dot = (x_tilde' * inv(A) * W_hat * (eye(size(Lambda)) - Lambda))' * x_hat_bar';
    

end

function sigma = activate(x)
    % sigma = tanh(x) + 2*ones(size(x));
    sigma = tanh(x);
end

== matlab function main_sim5/NN identification/NLPNN Learning Rule (1)/MATLAB Function3 ==
  data: e input; z input; z_dot output; lambda parameter
function z_dot = z_filter(e,z, lambda)


    z_dot = -lambda * z + e;

end

== matlab function main_sim5/NN identification/Momentum State1 ==
  data: x input; X output; m1 parameter; m2 parameter; l1 parameter; l2 parameter; lc1 parameter; lc2 parameter; I1 parameter; I2 parameter; I1m parameter; I2m parameter
function X = fcn(x, m1, m2, l1, l2, lc1, lc2, I1, I2, I1m, I2m)

    M = Inertia_M(x(1:2), x(3:4), m1, m2, l1, l2, lc1, lc2, I1, I2, I1m, I2m);
    
    X = [x(1:2); M * x(3:4)];

end



function M = Inertia_M(q, q_dot, m1, m2, l1, l2, lc1, lc2, I1, I2, I1m, I2m)
    %%
    q1 = q(1); q2 = q(2);
    q_dot1 = q_dot(1); q_dot2 = q_dot(2); 
  
    g = 9.81;    
    %%
    Mmat11=I1+I2+lc1^2*m1+l1^2*m2+lc2^2*m2+2*l1*lc2*m2*cos(q2) + I1m;
    Mmat12=I2+lc2^2*m2+l1*lc2*m2*cos(q2);
    Mmat21=I2+lc2^2*m2+l1*lc2*m2*cos(q2);
    Mmat22=I2+lc2^2*m2 + I2m;
    
    %%
    M = [
        Mmat11 Mmat12
        Mmat21 Mmat22  
        ];

end

== matlab function main_sim5/NN identification/Momentum State ==
  data: x input; X output; params parameter
function X = fcn(x, params)

    M = Inertia_M(x(1:2), x(3:4), params);

    X = [x(1:2); M * x(3:4)];

end



function M = Inertia_M(q, q_dot, params)
    m1 = params.m1;  m2 = params.m2;
    l1 = params.l1;  l2 = params.l2;
    lc1 = params.lc1;  lc2 = params.lc2;
    I1 = params.I1;  I2 = params.I2;
    I1m = params.I1m; I2m = params.I2m;
    b1 = params.b1;  b2 = params.b2;
    fc1 = params.fc1; fc2 = params.fc2;
    k1 = params.k1;  k2 = params.k2;    
    q1 = q(1); q2 = q(2);
    q_dot1 = q_dot(1); q_dot2 = q_dot(2); 
  
    g = 9.81;    
    %%
    Mmat11=I1+I2+lc1^2*m1+l1^2*m2+lc2^2*m2+2*l1*lc2*m2*cos(q2) + I1m;
    Mmat12=I2+lc2^2*m2+l1*lc2*m2*cos(q2);
    Mmat21=I2+lc2^2*m2+l1*lc2*m2*cos(q2);
    Mmat22=I2+lc2^2*m2 + I2m;
    
    %%
    M = [
        Mmat11 Mmat12
        Mmat21 Mmat22  
        ];

end

== matlab function main_sim5/NN identification/Subsystem/NN Learning Rule ==
  data: V_hat_dot output; W_hat_dot output; V_old input; W_old input; e input; x_hat_bar input; A parameter; n_h parameter; eta1 parameter; eta2 parameter; rho1 parameter; rho2 parameter
function [V_hat_dot, W_hat_dot] = learningrule(V_old, W_old, e, x_hat_bar, A, n_h, eta1, eta2, rho1, rho2)

    % J = 1/2 * integral(x_tilde' * x_tilde * dt)
    W_hat = W_old;
    V_hat = V_old;

    % identification
    x_tilde = e;

    % Lambda = zeros(n_h,n_h);
    Lambda = diag(tanh(V_hat * x_hat_bar).^2);

    % update the weights
    W_hat_dot = - eta1 * (x_tilde' * inv(A))' * activate(V_hat*x_hat_bar)' - rho1 * norm(x_tilde) * W_hat;
    V_hat_dot = - eta2 * (x_tilde' * inv(A) * W_hat * (eye(size(Lambda)) - Lambda))' * x_hat_bar' - rho2 * norm(x_tilde) * V_hat;


    % W_hat_dot = (x_tilde' * inv(A))' * activate(V_hat*x_hat_bar)';
    % V_hat_dot = (x_tilde' * inv(A) * W_hat * (eye(size(Lambda)) - Lambda))' * x_hat_bar';

    
end

function sigma = activate(x)
    % sigma = tanh(x) + 2*ones(size(x));
    sigma = tanh(x);
end

== matlab function main_sim5/NN identification/NN ==
  data: x_hat_bar input; g_hat output size=[4 1]; W_in input; W_out output; V_in input; V_out output; n_o parameter; n_i parameter; n_h parameter
function [g_hat,W_out,V_out] = NN(x_hat_bar, W_in,V_in, n_o, n_i, n_h)
    
    V_hat = V_in;
    W_hat = W_in;
    
    g_hat = W_hat * activate(V_hat * x_hat_bar);

    W_out = W_hat;
    V_out = V_hat;

end

function sigma = activate(x)
    sigma = tanh(x);
end

== matlab function main_sim5/Subsystem1/Inv Momentum State ==
  data: X input; x output; M input
function x = fcn(X, M)

    x = [X(1:2); M \ X(3:4)];

end

== matlab function main_sim5/Subsystem1/Inv Momentum State1 ==
  data: X input; x output; M input
function x = fcn(X, M)

    x = [X(1:2); M \ X(3:4)];

end
